simulink model "Model1_Current"  (R2023b)
settings: Solver=FixedStepAuto  StartTime=0.0  StopTime=Inf  FixedStep=1e-4  RelTol=1e-3
PostLoadFcn:
  | if any(exist('dsrtsu_mdlpostloadfcn', 'file') ~= 0), dsrtsu_mdlpostloadfcn('Execute', bdroot); end
InitFcn:
  | , if any(exist('rtifpga_mdlclblib', 'file') ~= 0), rtifpga_mdlclblib('Init', bdroot); end,
  | , if any(exist('dsmpb_private', 'file') ~= 0), dsmpb_private('dsmpb_mdlclblib', 'Init', bdroot); end,
  | load('LUT_BRUSA_jax_grad.mat')
  | load('daten_nichtlinear_interpoliert.mat')
  | load('Maschinendaten.mat')
  | load('PI_Controller.mat')
  | load('Nonlinear_IPMSM.mat')
values from neighbouring files (symbols this model uses):
  I_max = 170    [Maschinendaten.mat]    (also in Maschinendaten_Vorgabe.m; test_ModelParameters.m = evalin('base', 'I_max'); test_StrategySelection.m = tc.readConstant(tc.BLK_Imax))
  ID = [-250 -250 -250 -250 -250 -250 -250 -250 -250 -250 -250 -250 ... (10000 elements, 100x100)]    [daten_nichtlinear_interpoliert.mat]
  id_fine = linspace(min(id_vec), max(id_vec), 100)    [Messdaten_Interpoliert.m]    (also in daten_nichtlinear_interpoliert.mat = [-250 -247.474747475 -244.949494949 -242.424242424 -239.8989)
  IQ = [-250 -244.949494949 -239.898989899 -234.848484848 -229.797979798 -224.747474747 -219.696969697 -214.646464646 -209.595959596 -204.545454545 -199.494949495 -194.444444444 ... (10000 elements, 100x100)]    [daten_nichtlinear_interpoliert.mat]
  iq_fine = linspace(min(iq_vec), max(iq_vec), 100)    [Messdaten_Interpoliert.m]    (also in daten_nichtlinear_interpoliert.mat = [-250 -244.949494949 -239.898989899 -234.848484848 -229.7979)
  Ld = Ldd_fine    [Messdaten_Interpoliert.m]    (also in daten_nichtlinear_interpoliert.mat = [0.000225276031415 0.000225750625371 0.000226241749969 0.000)
  Lm = Lm_fine1    [Messdaten_Interpoliert.m]    (also in daten_nichtlinear_interpoliert.mat = [1.34827571578e-05 1.31035668506e-05 1.23153687442e-05 1.146)
  Lq = Lqq_fine    [Messdaten_Interpoliert.m]    (also in daten_nichtlinear_interpoliert.mat = [0.000286039721686 0.000286453471045 0.000286025480511 0.000)
  n_max = 11000    [Maschinendaten.mat]    (also in Maschinendaten_Vorgabe.m; test_ModelParameters.m = evalin('base', 'n_max'); test_StrategySelection.m = tc.readConstant(tc.BLK_nmax))
  p = 3    [Maschinendaten.mat]    (also in Maschinendaten_Vorgabe.m; Messdaten_Interpoliert.m; test_ModelParameters.m = evalin('base', 'p'))
  PSID = Psid_fine    [Messdaten_Interpoliert.m]    (also in daten_nichtlinear_interpoliert.mat = [0.00602681114795 0.00609490588107 0.00615917040906 0.006219)
  PSIQ = PSIQ1 - PSIQ1(iq0_idx,:)    [Messdaten_Interpoliert.m]    (also in daten_nichtlinear_interpoliert.mat = [-0.151946994742 -0.150499709177 -0.149057806808 -0.14762041)
  Rs = 0.018    [Maschinendaten.mat]    (also in Maschinendaten_Vorgabe.m; test_ModelParameters.m = evalin('base', 'Rs'))
  U_dc = 560    [Maschinendaten.mat]    (also in Maschinendaten_Vorgabe.m; test_ModelParameters.m = evalin('base', 'U_dc'))
  U_max = 323.316150746    [Maschinendaten.mat]    (also in Maschinendaten_Vorgabe.m = U_dc / sqrt(3); test_ModelParameters.m = evalin('base', 'U_max'))
libraries: dsmpblib x6
(part 2 of 2)

== matlab function Model1_Current/Subsystem Arbeitspunktsteuerung/Arbeitspunktsteuerung/Kennfelder/MTPV-Kennlinie ==
  data: Lm input; f_MTPV output; Ld input; Lq input; Lm2 input; Ld2 input; Lq2 input; Ldq input; Ldq_p input; Lq_d input; PSID input; PSIQ input; p input; omega2 input; ID input; IQ input; Rs2 input
%% MTPV Kennlinie 
% Ändert sich mit Drehzahl omega
function f_MTPV = fcn(Lm, Ld, Lq, Lm2, Ld2, Lq2, Ldq, Ldq_p, Lq_d, PSID, PSIQ, p, omega2, ID, IQ, Rs2)

Mv11 = omega2*Lm2.*(Ldq_p)...
       + (Ldq)./2 .*(Rs2 + omega2*(Ld2 + Lm2));
Mv12 = Lm./2.*(2*Rs2+omega2*(Ld2 + Lq2 + 2*Lm2));
Mv22 = omega2*Lm2.*(Ldq_p)...
       - (Ldq)./2 .*(Rs2 + omega2*(Lq2 + Lm2));
mv1 = 1.5*p*((Rs2 + omega2* (2*Ld2 - Lq_d + 3*Lm2)).*PSID./4 ... 
      + omega2*Lm.* (Ldq_p).*PSIQ./2);
mv2 = 1.5*p*(omega2*Lm.* (Ldq_p).*PSID./2 ...
      + (Rs2 + omega2*(2*Ld2 - Lq_d + 3*Lm2)).*PSIQ./4);
my_v = 0.75*p*omega2*(Ld.*(PSID).^2 + 2*Lm.*PSID.*PSIQ + Lq.*(PSIQ).^2);

f_MTPV = 1.5*p*(Mv11.*ID.^2 + 2*Mv12.*ID.*IQ + Mv22.*IQ.^2)...
         + 2*(mv1.*ID + mv2.*IQ) + my_v;
